simulink model "bo1808_svpwm_builtin"  (R2024b)
settings: Solver=ode23tb  StartTime=0.0  StopTime=t_stop_svpwm  MaxStep=Ts_sim_svpwm  RelTol=1e-3
undefined symbols (not defined in the file): omega_ref_svpwm, Uref_svpwm, Vdc
libraries: spsSVPWMGenerator2LevelLib x1
settings Model: Creator=26683  LastModifiedBy=26683

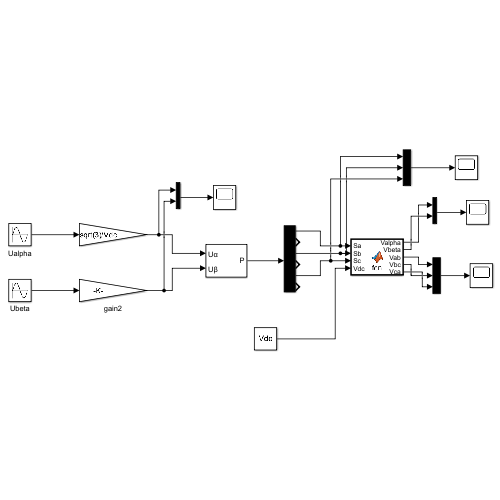
[thumbnail: Simulink's stored preview of the top-level diagram]
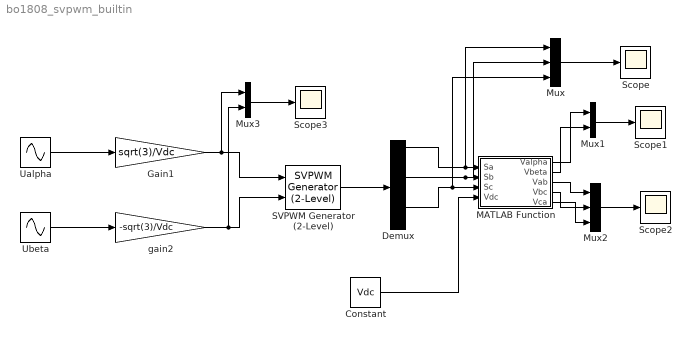
== system bo1808_svpwm_builtin ==
  Constant : Constant  Value=Vdc
  Demux : Demux  Outputs=6
  Gain1 : Gain  Gain=sqrt(3)/Vdc
  MATLAB Function : MATLAB Function  TreatAsAtomicUnit=on
  Mux : Mux  Inputs=3
  Mux1 : Mux  Inputs=2
  Mux2 : Mux  Inputs=3
  Mux3 : Mux  Inputs=2
  SVPWM Generator (2-Level) : spsSVPWMGenerator2LevelLib/SVPWM Generator (2-Level)  InputType=alpha-beta components  SwitchingPattern=Pattern #1  Fc=fs_pwm  ParUref=[0.8 -30 50]  Ts=0
  Scope{,1..3} (4 alike) : Scope
  Ualpha : Sin  Amplitude=Uref_svpwm  Frequency=omega_ref_svpwm  Phase=pi/2  SampleTime=0
  Ubeta : Sin  Amplitude=Uref_svpwm  Frequency=omega_ref_svpwm  SampleTime=0
  gain2 : Gain  Gain=-sqrt(3)/Vdc
  wires:
  Gain1/1 -> Mux3/1, SVPWM Generator (2-Level)/1
  gain2/1 -> Mux3/2, SVPWM Generator (2-Level)/2
  Constant/1 -> MATLAB Function/4(Vdc)
  Ualpha/1 -> Gain1/1
  Ubeta/1 -> gain2/1
  SVPWM Generator (2-Level)/1 -> Demux/1
  Demux/1 -> Mux/1, MATLAB Function/1(Sa)
  Demux/3 -> Mux/2, MATLAB Function/2(Sb)
  Demux/5 -> MATLAB Function/3(Sc), Mux/3
  Mux/1 -> Scope/1
  Mux1/1 -> Scope1/1
  MATLAB Function/1(Valpha) -> Mux1/1
  MATLAB Function/2(Vbeta) -> Mux1/2
  MATLAB Function/3(Vab) -> Mux2/1
  MATLAB Function/4(Vbc) -> Mux2/2
  MATLAB Function/5(Vca) -> Mux2/3
  Mux2/1 -> Scope2/1
  Mux3/1 -> Scope3/1

== matlab function bo1808_svpwm_builtin/MATLAB Function ==
  data: Sa input; Valpha output; Sb input; Sc input; Vdc input; Vbeta output; Vab output; Vbc output; Vca output
function [Valpha,Vbeta,Vab,Vbc,Vca] = fcn(Sa,Sb,Sc,Vdc)
sa = double(Sa);
sb = double(Sb);
sc = double(Sc);

Va0 = (sa - 0.5)*Vdc;
Vb0 = (sb - 0.5)*Vdc;
Vc0 = (sc - 0.5)*Vdc;

Vab = Va0 - Vb0;
Vbc = Vb0 - Vc0;
Vca = Vc0 - Va0;

Valpha = (2/3)*(Va0 - 0.5*Vb0 - 0.5*Vc0);
Vbeta  = (2/3)*(sqrt(3)/2)*(Vb0 - Vc0);
end
